simulink library "lib_fuel_converter3"  (Simulink 10.1)
settings: Solver=VariableStepAuto  StartTime=0.0  StopTime=10.0  RelTol=1e-3
undefined symbols (not defined in the file or in its folder): air_cp, amb_tmp, cyc_mph, ex_gas_cp, fc_acc_mass, fc_base_mass, fc_c2i_th_cond, fc_c_init_tmp, fc_cl2h_eff, fc_CO2_to_FUELgps, fc_cold, fc_cold_tmp, fc_cp, fc_ct_trq, fc_emisv, fc_ext_sarea, fc_fuel_den, fc_fuel_lhv, fc_h2x_th_cond, fc_h_air_flow, fc_h_cp, fc_h_init_tmp, fc_hood_emisv, fc_hood_sarea, fc_i2x_th_cond, fc_i_init_tmp, fc_inertia, fc_map_spd, fc_map_trq, fc_max_trq, fc_pwr_scale, fc_spd_scale, fc_trq_scale, fc_tstat, fc_x_init_tmp, fd_ratio, gb_num_init, gb_ratio, pow, vc_idle_bool, vc_idle_spd, vc_key_on, veh_glider_mass, wh_radius
undefined symbols (not defined in the file): fc_co_map, fc_co_map_c2h, fc_exflow_map, fc_extmp_map, fc_fuel_map, fc_fuel_map_c2h, fc_hc_map, fc_hc_map_c2h, fc_nn_model_name, fc_nox_map, fc_nox_map_c2h, fc_o2_map, fc_pm_map, fc_pm_map_c2h, generalName, logFlag
libraries: $bdroot x4, lib_etc x4, lib_fuel_converter x2, lib_fuel_converter2 x1
(part 3 of 8)

== system lib_fuel_converter3/fuel converter  <fc> for series/Model & Interface/model ==
  torque and speed  req'd at engine  output shaft (Nm) : Inport
  Block NOTES : Subsystem
      mask Display: disp('Block\nNOTES')
  Constant : Constant
  Demux : Demux  Outputs=2
  Demux1 : Demux  Outputs=3
  Logical Operator : Logic  Operator=NOT  Inputs=1
  Memory : Memory  InitialCondition=vc_idle_spd
  Mux : Mux  Inputs=2
  Mux1 : Mux  Inputs=2
  Selector : Selector  InputPortWidth=3  IndexOptions=Index vector (dialog)  Indices=[2]  OutputSizes=1
  Switch : Switch  Threshold=eps  SaturateOnIntegerOverflow=on  InputSameDT=on
  clutch disengaged : RelationalOperator  Operator===  RndMeth=Nearest  InputSameDT=on
  enhancedToWorkspace : Subsystem  TreatAsAtomicUnit=on  mask(enhancedToWorkspace){generalName=generalName, specificName=spd_out_r, logFlag=logFlag}
      mask prompts: generalName "General Name [char-evaluated]"; specificName "Specific Name [char-literal]"; logFlag "Enable flag (1=on,0=off)"
      mask help: A wrapper for the Simulink "To Workspace" block that allows you to evaluate the name of the variable to log to workspace. This is useful to avoid the double logging errors that occur when you pull in two library models that attempt to log to the same variable.
      mask init:
      | enhancedToWsMaker
      settings: CopyFcn=breakLinkCopyFcn  ParentCloseFcn=breakLinkParCloseFcn
      mask Help:
      | <h2>Enhanced To Workspace Block</h2>
      | <h3>Parameters</h3>
      | <UL>
      | <li><b>General Name:</b> This is the more general name of the variable. Variables are saved to the workspace as <i>generalName_specificName</i>. Note that this is an evaluated variable. If you would like to type in the value directly, it must be surrounded with single quotes. Otherwise you can input the name of a variable containing a char string.</li>
      | <li><b>Specific Name:</b> This is the specific name of the variable. Note that this is input as a char literal (i.e., you don't need quotes).</li>
      | <li><b>Enable Flag:</b> This flag should have the value of 0 or 1. If 0, the variable will not be logged to the workspace. If 1, the variable will be logged. This is done so that variable logging can be turned off to improve speed.</li>
      | </ul>
      | <h3>Overview</h3>
      | <p>The enhanced to workspace block was put together to allow one to dynamically resolve variable names at run time in simulink. This is most powerful when used in conjunction with a masked subsystem to allow multiple instances of that masked subsytem to be used in the same model. The strategy is to set the generalName in the block mask which will allow the block to change the general name for all variable logging on the fly.
      | <h3>Helper Files</h3>
      | <p>Three m-files are required by the enhancedToWorkspace block. These files are located in the &lt; ADVISOR root &gt;/GUI directory :
      | <ul>
      | <li><i>enhancedToWsMaker.m</i> This file runs the mask initialization for the block</li>
      | <li><i>breakLinkCopyFcn.m</i> This file is used by the block callback when the simulink block is copied. It is necessary to break the link to the enhancedToWorkspace similar to the To Workspace block in order for it to be able to configure itself. (Try copying simulink's To Workspace block--it is impossible to make a link)</li>
      | <li><i>breakLinkParCloseFcn.m</i> This file is similar to the breakLinkCopyFcn and is used when a parent system is closed</li>
      | </ul>
      | <hr>
      | 
      | <p>Created 2003-Jan-21, Michael Patrick O'Keefe, NREL</p>
      | 
      | <!--
      | <VARDEF>
      | <H3>var_name</H3>
      | <UL>
      | <LI><B>data type</B> data type here</LI>
      | <LI><B>units</B> units here</LI>
      | <LI><B>vehicle type</B> vehicle type here</LI>
      | <LI><B>description</B> description here</LI>
      | </UL>
      | </VARDEF>
      | -->
      mask Display: disp([generalName,'_',specificName])
  enhancedToWorkspace1 : Subsystem  TreatAsAtomicUnit=on  mask(enhancedToWorkspace){generalName=generalName, specificName=trq_out_r, logFlag=logFlag}
      mask prompts: generalName "General Name [char-evaluated]"; specificName "Specific Name [char-literal]"; logFlag "Enable flag (1=on,0=off)"
      mask help: A wrapper for the Simulink "To Workspace" block that allows you to evaluate the name of the variable to log to workspace. This is useful to avoid the double logging errors that occur when you pull in two library models that attempt to log to the same variable.
      mask init:
      | enhancedToWsMaker
      settings: CopyFcn=breakLinkCopyFcn  ParentCloseFcn=breakLinkParCloseFcn
      mask Help:
      | <h2>Enhanced To Workspace Block</h2>
      | <h3>Parameters</h3>
      | <UL>
      | <li><b>General Name:</b> This is the more general name of the variable. Variables are saved to the workspace as <i>generalName_specificName</i>. Note that this is an evaluated variable. If you would like to type in the value directly, it must be surrounded with single quotes. Otherwise you can input the name of a variable containing a char string.</li>
      | <li><b>Specific Name:</b> This is the specific name of the variable. Note that this is input as a char literal (i.e., you don't need quotes).</li>
      | <li><b>Enable Flag:</b> This flag should have the value of 0 or 1. If 0, the variable will not be logged to the workspace. If 1, the variable will be logged. This is done so that variable logging can be turned off to improve speed.</li>
      | </ul>
      | <h3>Overview</h3>
      | <p>The enhanced to workspace block was put together to allow one to dynamically resolve variable names at run time in simulink. This is most powerful when used in conjunction with a masked subsystem to allow multiple instances of that masked subsytem to be used in the same model. The strategy is to set the generalName in the block mask which will allow the block to change the general name for all variable logging on the fly.
      | <h3>Helper Files</h3>
      | <p>Three m-files are required by the enhancedToWorkspace block. These files are located in the &lt; ADVISOR root &gt;/GUI directory :
      | <ul>
      | <li><i>enhancedToWsMaker.m</i> This file runs the mask initialization for the block</li>
      | <li><i>breakLinkCopyFcn.m</i> This file is used by the block callback when the simulink block is copied. It is necessary to break the link to the enhancedToWorkspace similar to the To Workspace block in order for it to be able to configure itself. (Try copying simulink's To Workspace block--it is impossible to make a link)</li>
      | <li><i>breakLinkParCloseFcn.m</i> This file is similar to the breakLinkCopyFcn and is used when a parent system is closed</li>
      | </ul>
      | <hr>
      | 
      | <p>Created 2003-Jan-21, Michael Patrick O'Keefe, NREL</p>
      | 
      | <!--
      | <VARDEF>
      | <H3>var_name</H3>
      | <UL>
      | <LI><B>data type</B> data type here</LI>
      | <LI><B>units</B> units here</LI>
      | <LI><B>vehicle type</B> vehicle type here</LI>
      | <LI><B>description</B> description here</LI>
      | </UL>
      | </VARDEF>
      | -->
      mask Display: disp([generalName,'_',specificName])
  enhancedToWorkspace2 : Subsystem  TreatAsAtomicUnit=on  mask(enhancedToWorkspace){generalName=generalName, specificName=spd_est, logFlag=logFlag}
      mask prompts: generalName "General Name [char-evaluated]"; specificName "Specific Name [char-literal]"; logFlag "Enable flag (1=on,0=off)"
      mask help: A wrapper for the Simulink "To Workspace" block that allows you to evaluate the name of the variable to log to workspace. This is useful to avoid the double logging errors that occur when you pull in two library models that attempt to log to the same variable.
      mask init:
      | enhancedToWsMaker
      settings: CopyFcn=breakLinkCopyFcn  ParentCloseFcn=breakLinkParCloseFcn
      mask Help:
      | <h2>Enhanced To Workspace Block</h2>
      | <h3>Parameters</h3>
      | <UL>
      | <li><b>General Name:</b> This is the more general name of the variable. Variables are saved to the workspace as <i>generalName_specificName</i>. Note that this is an evaluated variable. If you would like to type in the value directly, it must be surrounded with single quotes. Otherwise you can input the name of a variable containing a char string.</li>
      | <li><b>Specific Name:</b> This is the specific name of the variable. Note that this is input as a char literal (i.e., you don't need quotes).</li>
      | <li><b>Enable Flag:</b> This flag should have the value of 0 or 1. If 0, the variable will not be logged to the workspace. If 1, the variable will be logged. This is done so that variable logging can be turned off to improve speed.</li>
      | </ul>
      | <h3>Overview</h3>
      | <p>The enhanced to workspace block was put together to allow one to dynamically resolve variable names at run time in simulink. This is most powerful when used in conjunction with a masked subsystem to allow multiple instances of that masked subsytem to be used in the same model. The strategy is to set the generalName in the block mask which will allow the block to change the general name for all variable logging on the fly.
      | <h3>Helper Files</h3>
      | <p>Three m-files are required by the enhancedToWorkspace block. These files are located in the &lt; ADVISOR root &gt;/GUI directory :
      | <ul>
      | <li><i>enhancedToWsMaker.m</i> This file runs the mask initialization for the block</li>
      | <li><i>breakLinkCopyFcn.m</i> This file is used by the block callback when the simulink block is copied. It is necessary to break the link to the enhancedToWorkspace similar to the To Workspace block in order for it to be able to configure itself. (Try copying simulink's To Workspace block--it is impossible to make a link)</li>
      | <li><i>breakLinkParCloseFcn.m</i> This file is similar to the breakLinkCopyFcn and is used when a parent system is closed</li>
      | </ul>
      | <hr>
      | 
      | <p>Created 2003-Jan-21, Michael Patrick O'Keefe, NREL</p>
      | 
      | <!--
      | <VARDEF>
      | <H3>var_name</H3>
      | <UL>
      | <LI><B>data type</B> data type here</LI>
      | <LI><B>units</B> units here</LI>
      | <LI><B>vehicle type</B> vehicle type here</LI>
      | <LI><B>description</B> description here</LI>
      | </UL>
      | </VARDEF>
      | -->
      mask Display: disp([generalName,'_',specificName])
  enhancedToWorkspace3 : Subsystem  TreatAsAtomicUnit=on  mask(enhancedToWorkspace){generalName=generalName, specificName=brake_trq, logFlag=logFlag}
      mask prompts: generalName "General Name [char-evaluated]"; specificName "Specific Name [char-literal]"; logFlag "Enable flag (1=on,0=off)"
      mask help: A wrapper for the Simulink "To Workspace" block that allows you to evaluate the name of the variable to log to workspace. This is useful to avoid the double logging errors that occur when you pull in two library models that attempt to log to the same variable.
      mask init:
      | enhancedToWsMaker
      settings: CopyFcn=breakLinkCopyFcn  ParentCloseFcn=breakLinkParCloseFcn
      mask Help:
      | <h2>Enhanced To Workspace Block</h2>
      | <h3>Parameters</h3>
      | <UL>
      | <li><b>General Name:</b> This is the more general name of the variable. Variables are saved to the workspace as <i>generalName_specificName</i>. Note that this is an evaluated variable. If you would like to type in the value directly, it must be surrounded with single quotes. Otherwise you can input the name of a variable containing a char string.</li>
      | <li><b>Specific Name:</b> This is the specific name of the variable. Note that this is input as a char literal (i.e., you don't need quotes).</li>
      | <li><b>Enable Flag:</b> This flag should have the value of 0 or 1. If 0, the variable will not be logged to the workspace. If 1, the variable will be logged. This is done so that variable logging can be turned off to improve speed.</li>
      | </ul>
      | <h3>Overview</h3>
      | <p>The enhanced to workspace block was put together to allow one to dynamically resolve variable names at run time in simulink. This is most powerful when used in conjunction with a masked subsystem to allow multiple instances of that masked subsytem to be used in the same model. The strategy is to set the generalName in the block mask which will allow the block to change the general name for all variable logging on the fly.
      | <h3>Helper Files</h3>
      | <p>Three m-files are required by the enhancedToWorkspace block. These files are located in the &lt; ADVISOR root &gt;/GUI directory :
      | <ul>
      | <li><i>enhancedToWsMaker.m</i> This file runs the mask initialization for the block</li>
      | <li><i>breakLinkCopyFcn.m</i> This file is used by the block callback when the simulink block is copied. It is necessary to break the link to the enhancedToWorkspace similar to the To Workspace block in order for it to be able to configure itself. (Try copying simulink's To Workspace block--it is impossible to make a link)</li>
      | <li><i>breakLinkParCloseFcn.m</i> This file is similar to the breakLinkCopyFcn and is used when a parent system is closed</li>
      | </ul>
      | <hr>
      | 
      | <p>Created 2003-Jan-21, Michael Patrick O'Keefe, NREL</p>
      | 
      | <!--
      | <VARDEF>
      | <H3>var_name</H3>
      | <UL>
      | <LI><B>data type</B> data type here</LI>
      | <LI><B>units</B> units here</LI>
      | <LI><B>vehicle type</B> vehicle type here</LI>
      | <LI><B>description</B> description here</LI>
      | </UL>
      | </VARDEF>
      | -->
      mask Display: disp([generalName,'_',specificName])
  fuel use and EO emis Configurable Subsystem : Subsystem  BlockChoice=fuel use and EO emis
      link override fuel use and EO emis/enhancedToWorkspace1/To Workspace: VariableName=fc_th_pwr  SampleTime=-1  SaveFormat=Array
      link override fuel use and EO emis/enhancedToWorkspace10/To Workspace: VariableName=fc_ex_gas_tmp  SampleTime=-1  SaveFormat=Array
      link override fuel use and EO emis/enhancedToWorkspace11/To Workspace: VariableName=fc_ex_th_pwr  SampleTime=-1  SaveFormat=Array
      link override fuel use and EO emis/enhancedToWorkspace12/To Workspace: VariableName=fc_clt_tmp  SampleTime=-1  SaveFormat=Array
      link override fuel use and EO emis/enhancedToWorkspace2/To Workspace: VariableName=fc_o2_flow  SampleTime=-1  SaveFormat=Array
      link override fuel use and EO emis/enhancedToWorkspace3/To Workspace: VariableName=fc_r_th_pwr  SampleTime=-1  SaveFormat=Array
      link override fuel use and EO emis/enhancedToWorkspace5/To Workspace: VariableName=fc_h_th_pwr  SampleTime=-1  SaveFormat=Array
      link override fuel use and EO emis/enhancedToWorkspace6/To Workspace: VariableName=fc_tmp  SampleTime=-1  SaveFormat=Array
      link override fuel use and EO emis/enhancedToWorkspace7/To Workspace: VariableName=fc_fuel_rate  SampleTime=-1  SaveFormat=Array
      link override fuel use and EO emis/enhancedToWorkspace8/To Workspace: VariableName=fc_emis_eo  SampleTime=-1  SaveFormat=Array
      link override fuel use and EO emis/enhancedToWorkspace9/To Workspace: VariableName=fc_ex_gas_flow  SampleTime=-1  SaveFormat=Array
      settings: AttributesFormatString=%<BlockChoice>  TemplateBlock=lib_fuel_converter3/configurable subsystems/fuel use and EO emis Configurable Subsystem  MemberBlocks=fuel use and EO emis,fuel use and EO emis Neural Network Model
  help : Subsystem
      settings: OpenFcn=web(['file:\\\' which('fuel_converter.htm')]);
      mask Display: image(imread('doc_man.jpg'))
  providing trq (+ive or -ive) : Subsystem
  spinning up or spinning down : Subsystem
  fuel use : Outport  InitialOutput=0
  EO emis info : Outport  Port=2  InitialOutput=0
  "torque and speed  avail. to driveline (Nm), (rad/s)" : Outport  Port=3  InitialOutput=0
  tag scope: engine_speed=scoped, fc_brake_trq=scoped, fc_spd_est=scoped, fc_spd_out_a=scoped, fc_spd_out_r=scoped, fc_trq_out_a=scoped, fc_trq_out_r=scoped, fuel=scoped
  wires:
  Selector/1 -> [fc_spd_est], enhancedToWorkspace2/1(In1)
  fuel use and EO emis Configurable Subsystem/1(cumulative fuel  use (gal)) -> [fuel], fuel use/1
  Switch/1 -> Demux1/1
  Memory/1 -> providing trq (+ive or -ive)/3(prev engine spd (rad/s)), spinning up or spinning down/3(previous engine spd (rad/s))
  spinning up or spinning down/1(map trq (Nm) spd (rad/s) trq to drivetrain (Nm)) -> Switch/3
  providing trq (+ive or -ive)/1(map trq (Nm) spd (rad/s) trq to drivetrain (Nm)) -> Selector/1, Switch/1
  Logical Operator/1 -> Switch/2
  [clutch_state] -> clutch disengaged/2
  Constant/1 -> clutch disengaged/1
  clutch disengaged/1 -> Logical Operator/1, spinning up or spinning down/2(engine disconnected from drivetrain)
  Demux/2 -> [fc_spd_out_r], enhancedToWorkspace/1(In1), spinning up or spinning down/1(spd command (rad/s)), providing trq (+ive or -ive)/2(req'd spd (rad/s))
  Demux/1 -> providing trq (+ive or -ive)/1(req'd trq (Nm)), [fc_trq_out_r], enhancedToWorkspace1/1(In1)
  torque and speed  req'd at engine  output shaft (Nm)/1 -> Demux/1
  Demux1/1 -> fuel use and EO emis Configurable Subsystem/1(T (Nm)), [fc_brake_trq], enhancedToWorkspace3/1(In1)
  Demux1/3 -> [fc_trq_out_a], Mux1/1
  Demux1/2 -> fuel use and EO emis Configurable Subsystem/2(w (rad/s)), Mux1/2, Memory/1, [fc_spd_out_a], [engine_speed]
  Mux/1 -> EO emis info/1
  fuel use and EO emis Configurable Subsystem/2("FC ON?, EOem, MFex, Tex, O2ex") -> Mux/1
  fuel use and EO emis Configurable Subsystem/3(Vv,Tfc) -> Mux/2
  Mux1/1 -> "torque and speed  avail. to driveline (Nm), (rad/s)"/1

== system lib_fuel_converter3/fuel converter  <fc> for series/Model & Interface/signal annotator ==
  In1 : Inport
  Demux : Demux  Outputs=2
  Mux : Mux  Inputs=2
  Out1 : Outport
  wires:
  Mux/1 -> Out1/1
  In1/1 -> Demux/1
  Demux/1 -> Mux/1  "fc_trq_out_r"
  Demux/2 -> Mux/2  "fc_spd_out_r"

== system lib_fuel_converter3/fuel converter <fc>/IC Engine Model  &  Interface/ic engine model ==
  torque and speed  req'd at engine  output shaft (Nm) : Inport
  Block NOTES : Subsystem
      mask Display: disp('Block\nNOTES')
  Demux : Demux  Outputs=2
  Mux : Mux  Inputs=2
  Mux1 : Mux  Inputs=2
  Speed Limits : Subsystem
  engine speed estimator : Subsystem
  engine torque : Subsystem
  enhancedToWorkspace : Subsystem  mask(enhancedToWorkspace){generalName=generalName, specificName=spd_out_r, logFlag=logFlag}
      mask prompts: generalName "General Name [char-evaluated]"; specificName "Specific Name [char-literal]"; logFlag "Enable flag (1=on,0=off)"
      mask help: A wrapper for the Simulink "To Workspace" block that allows you to evaluate the name of the variable to log to workspace. This is useful to avoid the double logging errors that occur when you pull in two library models that attempt to log to the same variable.
      mask init:
      | enhancedToWsMaker
      settings: CopyFcn=breakLinkCopyFcn
      mask Display: disp([generalName,'_',specificName])
  enhancedToWorkspace1 : Subsystem  mask(enhancedToWorkspace){generalName=generalName, specificName=spd_est, logFlag=logFlag}
      mask prompts: generalName "General Name [char-evaluated]"; specificName "Specific Name [char-literal]"; logFlag "Enable flag (1=on,0=off)"
      mask help: A wrapper for the Simulink "To Workspace" block that allows you to evaluate the name of the variable to log to workspace. This is useful to avoid the double logging errors that occur when you pull in two library models that attempt to log to the same variable.
      mask init:
      | enhancedToWsMaker
      settings: CopyFcn=breakLinkCopyFcn
      mask Display: disp([generalName,'_',specificName])
  enhancedToWorkspace3 : Subsystem  mask(enhancedToWorkspace){generalName=generalName, specificName=fuel, logFlag=logFlag}
      mask prompts: generalName "General Name [char-evaluated]"; specificName "Specific Name [char-literal]"; logFlag "Enable flag (1=on,0=off)"
      mask help: A wrapper for the Simulink "To Workspace" block that allows you to evaluate the name of the variable to log to workspace. This is useful to avoid the double logging errors that occur when you pull in two library models that attempt to log to the same variable.
      mask init:
      | enhancedToWsMaker
      settings: CopyFcn=breakLinkCopyFcn
      mask Display: disp([generalName,'_',specificName])
  enhancedToWorkspace4 : Subsystem  mask(enhancedToWorkspace){generalName=generalName, specificName=spd_out_a, logFlag=logFlag}
      mask prompts: generalName "General Name [char-evaluated]"; specificName "Specific Name [char-literal]"; logFlag "Enable flag (1=on,0=off)"
      mask help: A wrapper for the Simulink "To Workspace" block that allows you to evaluate the name of the variable to log to workspace. This is useful to avoid the double logging errors that occur when you pull in two library models that attempt to log to the same variable.
      mask init:
      | enhancedToWsMaker
      settings: CopyFcn=breakLinkCopyFcn
      mask Display: disp([generalName,'_',specificName])
  enhancedToWorkspace5 : Subsystem  mask(enhancedToWorkspace){generalName=generalName, specificName=trq_out_a, logFlag=logFlag}
      mask prompts: generalName "General Name [char-evaluated]"; specificName "Specific Name [char-literal]"; logFlag "Enable flag (1=on,0=off)"
      mask help: A wrapper for the Simulink "To Workspace" block that allows you to evaluate the name of the variable to log to workspace. This is useful to avoid the double logging errors that occur when you pull in two library models that attempt to log to the same variable.
      mask init:
      | enhancedToWsMaker
      settings: CopyFcn=breakLinkCopyFcn
      mask Display: disp([generalName,'_',specificName])
  enhancedToWorkspace6 : Subsystem  mask(enhancedToWorkspace){generalName=generalName, specificName=trq_out_r, logFlag=logFlag}
      mask prompts: generalName "General Name [char-evaluated]"; specificName "Specific Name [char-literal]"; logFlag "Enable flag (1=on,0=off)"
      mask help: A wrapper for the Simulink "To Workspace" block that allows you to evaluate the name of the variable to log to workspace. This is useful to avoid the double logging errors that occur when you pull in two library models that attempt to log to the same variable.
      mask init:
      | enhancedToWsMaker
      settings: CopyFcn=breakLinkCopyFcn
      mask Display: disp([generalName,'_',specificName])
  enhancedToWorkspace7 : Subsystem  mask(enhancedToWorkspace){generalName=generalName, specificName=brake_trq, logFlag=logFlag}
      mask prompts: generalName "General Name [char-evaluated]"; specificName "Specific Name [char-literal]"; logFlag "Enable flag (1=on,0=off)"
      mask help: A wrapper for the Simulink "To Workspace" block that allows you to evaluate the name of the variable to log to workspace. This is useful to avoid the double logging errors that occur when you pull in two library models that attempt to log to the same variable.
      mask init:
      | enhancedToWsMaker
      settings: CopyFcn=breakLinkCopyFcn
      mask Display: disp([generalName,'_',specificName])
  fuel use and EO emis Configurable Subsystem : Subsystem  BlockChoice=fuel use and EO emis
      link override fuel use and EO emis/enhancedToWorkspace1/To Workspace: VariableName=fc_th_pwr  SampleTime=-1  SaveFormat=Array
      link override fuel use and EO emis/enhancedToWorkspace10/To Workspace: VariableName=fc_ex_gas_tmp  SampleTime=-1  SaveFormat=Array
      link override fuel use and EO emis/enhancedToWorkspace11/To Workspace: VariableName=fc_ex_th_pwr  SampleTime=-1  SaveFormat=Array
      link override fuel use and EO emis/enhancedToWorkspace12/To Workspace: VariableName=fc_clt_tmp  SampleTime=-1  SaveFormat=Array
      link override fuel use and EO emis/enhancedToWorkspace2/To Workspace: VariableName=fc_o2_flow  SampleTime=-1  SaveFormat=Array
      link override fuel use and EO emis/enhancedToWorkspace3/To Workspace: VariableName=fc_r_th_pwr  SampleTime=-1  SaveFormat=Array
      link override fuel use and EO emis/enhancedToWorkspace5/To Workspace: VariableName=fc_h_th_pwr  SampleTime=-1  SaveFormat=Array
      link override fuel use and EO emis/enhancedToWorkspace6/To Workspace: VariableName=fc_tmp  SampleTime=-1  SaveFormat=Array
      link override fuel use and EO emis/enhancedToWorkspace7/To Workspace: VariableName=fc_fuel_rate  SampleTime=-1  SaveFormat=Array
      link override fuel use and EO emis/enhancedToWorkspace8/To Workspace: VariableName=fc_emis_eo  SampleTime=-1  SaveFormat=Array
      link override fuel use and EO emis/enhancedToWorkspace9/To Workspace: VariableName=fc_ex_gas_flow  SampleTime=-1  SaveFormat=Array
      settings: AttributesFormatString=%<BlockChoice>  TemplateBlock=lib_fuel_converter3/configurable subsystems/fuel use and EO emis Configurable Subsystem  MemberBlocks=fuel use and EO emis,fuel use and EO emis Neural Network Model
  help : Subsystem
      settings: OpenFcn=web(['file:\\\' which('fuel_converter.htm')]);
      mask Display: image(imread('doc_man.jpg'))
  fuel use : Outport  InitialOutput=0
  EO emis info : Outport  Port=2  InitialOutput=0
  "torque and speed  avail. to driveline (Nm), (rad/s)" : Outport  Port=3  InitialOutput=0
  tag scope: fc_spd_est=scoped, fc_spd_out_a=scoped, fc_spd_out_r=scoped, fc_trq_out_a=scoped, fuel=scoped
  wires:
  engine torque/2(torque to shaft (Nm)) -> [fc_trq_out_a], Mux1/1, enhancedToWorkspace5/1(In1)
  engine torque/1(map torque (Nm)) -> enhancedToWorkspace7/1(In1), fuel use and EO emis Configurable Subsystem/1(T (Nm))
  Mux1/1 -> "torque and speed  avail. to driveline (Nm), (rad/s)"/1
  fuel use and EO emis Configurable Subsystem/3(Vv,Tfc) -> Mux/2
  fuel use and EO emis Configurable Subsystem/2("FC ON?, EOem, MFex, Tex, O2ex") -> Mux/1
  Mux/1 -> EO emis info/1
  Demux/1 -> engine torque/1(fc_trq_out_r), enhancedToWorkspace6/1(In1)
  torque and speed  req'd at engine  output shaft (Nm)/1 -> Demux/1
  Demux/2 -> Speed Limits/1(Speed Requested), [fc_spd_out_r], enhancedToWorkspace/1(In1)
  fuel use and EO emis Configurable Subsystem/1(cumulative fuel  use (gal)) -> fuel use/1, [fuel], enhancedToWorkspace3/1(In1)
  engine speed estimator/1(Out1) -> engine torque/3(engine spd), fuel use and EO emis Configurable Subsystem/2(w (rad/s)), [fc_spd_est], enhancedToWorkspace1/1(In1)
  Speed Limits/1(Limited Speed Request) -> engine torque/2(spd command), engine speed estimator/1(spd command), Mux1/2, [fc_spd_out_a], enhancedToWorkspace4/1(In1)

== system lib_fuel_converter3/fuel converter <fc>/IC Engine Model  &  Interface/signal annotator ==
  In1 : Inport
  Demux : Demux  Outputs=2
  Mux : Mux  Inputs=1
  Terminator : Terminator
  Out1 : Outport
  tag scope: fc_trq_out_r=scoped
  wires:
  Mux/1 -> Out1/1
  [fc_spd_est] -> Mux/1  "fc_spd_est"
  In1/1 -> Demux/1
  Demux/1 -> [fc_trq_out_r]  "fc_trq_out_r"
  Demux/2 -> Terminator/1  "fc_spd_out_r"

== system lib_fuel_converter3/fuel converter <fc> no fuel at negative torque/IC Engine Model  &  Interface/ic engine model ==
  torque and speed  req'd at engine  output shaft (Nm) : Inport
  Block NOTES : Subsystem
      mask Display: disp('Block\nNOTES')
  Demux : Demux  Outputs=2
  Demux1 : Demux  Outputs=2
  Demux2 : Demux  Outputs=2
  Mux : Mux  Inputs=2
  Mux1 : Mux  Inputs=2
  Speed Limits : Subsystem
  achieved power and energy : Subsystem
  engine speed estimator : Subsystem
  engine torque : Subsystem
  enhancedToWorkspace : Subsystem  mask(enhancedToWorkspace){generalName=generalName, specificName=spd_out_r, logFlag=logFlag}
      mask prompts: generalName "General Name [char-evaluated]"; specificName "Specific Name [char-literal]"; logFlag "Enable flag (1=on,0=off)"
      mask help: A wrapper for the Simulink "To Workspace" block that allows you to evaluate the name of the variable to log to workspace. This is useful to avoid the double logging errors that occur when you pull in two library models that attempt to log to the same variable.
      mask init:
      | enhancedToWsMaker
      settings: CopyFcn=breakLinkCopyFcn
      mask Display: disp([generalName,'_',specificName])
  enhancedToWorkspace1 : Subsystem  mask(enhancedToWorkspace){generalName=generalName, specificName=spd_est, logFlag=logFlag}
      mask prompts: generalName "General Name [char-evaluated]"; specificName "Specific Name [char-literal]"; logFlag "Enable flag (1=on,0=off)"
      mask help: A wrapper for the Simulink "To Workspace" block that allows you to evaluate the name of the variable to log to workspace. This is useful to avoid the double logging errors that occur when you pull in two library models that attempt to log to the same variable.
      mask init:
      | enhancedToWsMaker
      settings: CopyFcn=breakLinkCopyFcn
      mask Display: disp([generalName,'_',specificName])
  enhancedToWorkspace3 : Subsystem  mask(enhancedToWorkspace){generalName=generalName, specificName=fuel, logFlag=logFlag}
      mask prompts: generalName "General Name [char-evaluated]"; specificName "Specific Name [char-literal]"; logFlag "Enable flag (1=on,0=off)"
      mask help: A wrapper for the Simulink "To Workspace" block that allows you to evaluate the name of the variable to log to workspace. This is useful to avoid the double logging errors that occur when you pull in two library models that attempt to log to the same variable.
      mask init:
      | enhancedToWsMaker
      settings: CopyFcn=breakLinkCopyFcn
      mask Display: disp([generalName,'_',specificName])
  enhancedToWorkspace4 : Subsystem  mask(enhancedToWorkspace){generalName=generalName, specificName=spd_out_a, logFlag=logFlag}
      mask prompts: generalName "General Name [char-evaluated]"; specificName "Specific Name [char-literal]"; logFlag "Enable flag (1=on,0=off)"
      mask help: A wrapper for the Simulink "To Workspace" block that allows you to evaluate the name of the variable to log to workspace. This is useful to avoid the double logging errors that occur when you pull in two library models that attempt to log to the same variable.
      mask init:
      | enhancedToWsMaker
      settings: CopyFcn=breakLinkCopyFcn
      mask Display: disp([generalName,'_',specificName])
  enhancedToWorkspace5 : Subsystem  mask(enhancedToWorkspace){generalName=generalName, specificName=trq_out_a, logFlag=logFlag}
      mask prompts: generalName "General Name [char-evaluated]"; specificName "Specific Name [char-literal]"; logFlag "Enable flag (1=on,0=off)"
      mask help: A wrapper for the Simulink "To Workspace" block that allows you to evaluate the name of the variable to log to workspace. This is useful to avoid the double logging errors that occur when you pull in two library models that attempt to log to the same variable.
      mask init:
      | enhancedToWsMaker
      settings: CopyFcn=breakLinkCopyFcn
      mask Display: disp([generalName,'_',specificName])
  enhancedToWorkspace6 : Subsystem  mask(enhancedToWorkspace){generalName=generalName, specificName=trq_out_r, logFlag=logFlag}
      mask prompts: generalName "General Name [char-evaluated]"; specificName "Specific Name [char-literal]"; logFlag "Enable flag (1=on,0=off)"
      mask help: A wrapper for the Simulink "To Workspace" block that allows you to evaluate the name of the variable to log to workspace. This is useful to avoid the double logging errors that occur when you pull in two library models that attempt to log to the same variable.
      mask init:
      | enhancedToWsMaker
      settings: CopyFcn=breakLinkCopyFcn
      mask Display: disp([generalName,'_',specificName])
  enhancedToWorkspace7 : Subsystem  mask(enhancedToWorkspace){generalName=generalName, specificName=brake_trq, logFlag=logFlag}
      mask prompts: generalName "General Name [char-evaluated]"; specificName "Specific Name [char-literal]"; logFlag "Enable flag (1=on,0=off)"
      mask help: A wrapper for the Simulink "To Workspace" block that allows you to evaluate the name of the variable to log to workspace. This is useful to avoid the double logging errors that occur when you pull in two library models that attempt to log to the same variable.
      mask init:
      | enhancedToWsMaker
      settings: CopyFcn=breakLinkCopyFcn
      mask Display: disp([generalName,'_',specificName])
  fuel use and EO emis no fuel used at negative torque : Subsystem
  help : Subsystem
      settings: OpenFcn=web(['file:\\\' which('fuel_converter.htm')]);
      mask Display: image(imread('doc_man.jpg'))
  requested power and energy : Subsystem
  fuel use : Outport  InitialOutput=0
  EO emis info : Outport  Port=2  InitialOutput=0
  "torque and speed  avail. to driveline (Nm), (rad/s)" : Outport  Port=3  InitialOutput=0
  tag scope: fc_spd_est=scoped, fc_spd_out_a=scoped, fc_spd_out_r=scoped, fc_trq_out_a=scoped, fuel=scoped
  wires:
  engine torque/2(torque to shaft (Nm)) -> [fc_trq_out_a], Mux1/1, enhancedToWorkspace5/1(In1)
  engine torque/1(map torque (Nm)) -> enhancedToWorkspace7/1(In1), fuel use and EO emis no fuel used at negative torque/1(T (Nm))
  Mux1/1 -> "torque and speed  avail. to driveline (Nm), (rad/s)"/1, Demux2/1
  fuel use and EO emis no fuel used at negative torque/3(Vv,Tfc) -> Mux/2
  fuel use and EO emis no fuel used at negative torque/2("FC ON?, EOem, MFex, Tex, O2ex") -> Mux/1
  Mux/1 -> EO emis info/1
  Demux/1 -> engine torque/1(fc_trq_out_r), enhancedToWorkspace6/1(In1)
  torque and speed  req'd at engine  output shaft (Nm)/1 -> Demux/1, Demux1/1
  Demux/2 -> Speed Limits/1(Speed Requested), [fc_spd_out_r], enhancedToWorkspace/1(In1)
  fuel use and EO emis no fuel used at negative torque/1(cumulative fuel  use (gal)) -> fuel use/1, [fuel], enhancedToWorkspace3/1(In1)
  engine speed estimator/1(Out1) -> engine torque/3(engine spd), fuel use and EO emis no fuel used at negative torque/2(w (rad/s)), [fc_spd_est], enhancedToWorkspace1/1(In1)
  Speed Limits/1(Limited Speed Request) -> engine torque/2(spd command), engine speed estimator/1(spd command), Mux1/2, [fc_spd_out_a], enhancedToWorkspace4/1(In1)
  Demux1/1 -> requested power and energy/1(trq)
  Demux1/2 -> requested power and energy/2(spd)
  Demux2/1 -> achieved power and energy/1(trq)
  Demux2/2 -> achieved power and energy/2(spd)

== system lib_fuel_converter3/fuel converter <fc> no fuel at negative torque/IC Engine Model  &  Interface/signal annotator ==
  In1 : Inport
  Demux : Demux  Outputs=2
  Mux : Mux  Inputs=3
  Out1 : Outport
  wires:
  [fc_spd_est] -> Mux/3  "fc_spd_est"
  In1/1 -> Demux/1
  Demux/1 -> Mux/1  "fc_trq_out_r"
  Demux/2 -> Mux/2  "fc_spd_out_r"
  Mux/1 -> Out1/1

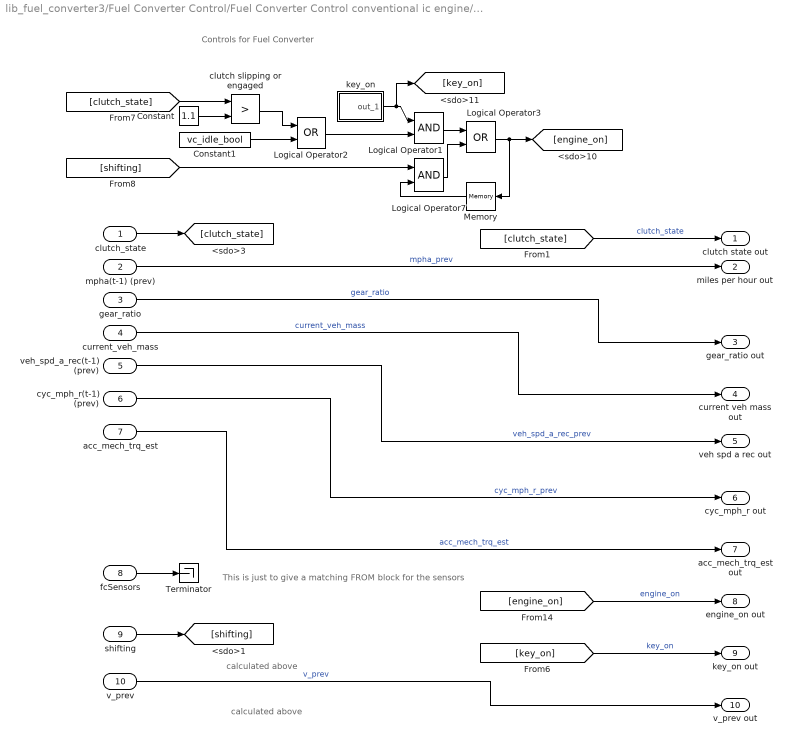
== system lib_fuel_converter3/Fuel Converter Control/Fuel Converter Control conventional ic engine/conventional IC engine/Fuel Converter Control ==
  note: Controls for Fuel Converter
  note: This is just to give a matching FROM block for the sensors
  note: calculated above
  note: calculated above
  clutch_state : Inport
  mpha(t-1) (prev) : Inport  Port=2
  gear_ratio : Inport  Port=3
  current_veh_mass : Inport  Port=4
  veh_spd_a_rec(t-1) (prev) : Inport  Port=5
  cyc_mph_r(t-1) (prev) : Inport  Port=6
  acc_mech_trq_est : Inport  Port=7
  fcSensors : Inport  Port=8
  shifting : Inport  Port=9
  v_prev : Inport  Port=10
  Constant : Constant  Value=1.1
  Constant1 : Constant  Value=vc_idle_bool
  Logical Operator1 : Logic
  Logical Operator2 : Logic  Operator=OR
  Logical Operator3 : Logic  Operator=OR
  Logical Operator7 : Logic
  Memory : Memory
  Terminator : Terminator
  clutch slipping or engaged : RelationalOperator  Operator=>  RndMeth=Nearest  InputSameDT=on
  key_on : Subsystem  mask(Repeating table){Parameter1=vc_key_on(:,1), Parameter2=vc_key_on(:,2)}
      mask prompts: Parameter1 "Time values:"; Parameter2 "Output values:"
      mask help:
      | Repeating table.
      | Enter values of time and output for first cycle.
      mask init:
      | period = max(@1); t = @1; y = @2;
      mask Help: Repeats cycle given in table. Time values should be monotonically increasing.
  clutch state out : Outport
  miles per hour out : Outport  Port=2
  gear_ratio out : Outport  Port=3
  current veh mass out : Outport  Port=4
  veh spd a rec out : Outport  Port=5
  cyc_mph_r out : Outport  Port=6
  acc_mech_trq_est out : Outport  Port=7
  engine_on out : Outport  Port=8
  key_on out : Outport  Port=9
  v_prev out : Outport  Port=10
  wires:
  gear_ratio/1 -> gear_ratio out/1  "gear_ratio"
  [clutch_state] -> clutch slipping or engaged/1
  Constant1/1 -> Logical Operator2/2
  Constant/1 -> clutch slipping or engaged/2
  clutch slipping or engaged/1 -> Logical Operator2/1
  Logical Operator1/1 -> Logical Operator3/1
  Logical Operator2/1 -> Logical Operator1/2
  [shifting] -> Logical Operator7/1
  Memory/1 -> Logical Operator7/2
  Logical Operator7/1 -> Logical Operator3/2
  Logical Operator3/1 -> [engine_on], Memory/1
  key_on/1(out_1) -> Logical Operator1/1, [key_on]
  fcSensors/1 -> Terminator/1
  shifting/1 -> [shifting]
  clutch_state/1 -> [clutch_state]
  mpha(t-1) (prev)/1 -> miles per hour out/1  "mpha_prev"
  current_veh_mass/1 -> current veh mass out/1  "current_veh_mass"
  veh_spd_a_rec(t-1) (prev)/1 -> veh spd a rec out/1  "veh_spd_a_rec_prev"
  cyc_mph_r(t-1) (prev)/1 -> cyc_mph_r out/1  "cyc_mph_r_prev"
  acc_mech_trq_est/1 -> acc_mech_trq_est out/1  "acc_mech_trq_est"
  v_prev/1 -> v_prev out/1  "v_prev"
  [clutch_state] -> clutch state out/1  "clutch_state"
  [engine_on] -> engine_on out/1  "engine_on"
  [key_on] -> key_on out/1  "key_on"

== system lib_fuel_converter3/configurable subsystems/fuel use and EO emis/HOT engine maps/Block NOTES ==
  note: This block determines the fully hot fuel use, engine-out emissions output rates, exhaust gas mass flow rate,
      | and engine-out exhaust gas temperature as a function of engine output torque and speed.
      | The engine maps (except for exhaust gas temperature) can be scaled using variables fc_spd_scale and
      |  fc_trq_scale; it is recommended that scaling values outside the range of 0.85 to 1.15 be used CAREFULLY.

== system lib_fuel_converter3/configurable subsystems/fuel use and EO emis/HOT engine maps/CO (g/s) ==
  x0 : Inport
  y0 : Inport  Port=2
  Mux : Mux  Inputs=2
  S-function : S-Function  FunctionName=sftable2  Parameters=xindex, yindex, table  SFunctionDeploymentMode=off  EnableBusSupport=off
  table out : Outport  InitialOutput=0
  wires:
  y0/1 -> Mux/2
  S-function/1 -> table out/1
  x0/1 -> Mux/1
  Mux/1 -> S-function/1

== system lib_fuel_converter3/configurable subsystems/fuel use and EO emis/HOT engine maps/HC (g/s) ==
  x0 : Inport
  y0 : Inport  Port=2
  Mux : Mux  Inputs=2
  S-function : S-Function  FunctionName=sftable2  Parameters=xindex, yindex, table  SFunctionDeploymentMode=off  EnableBusSupport=off
  table out : Outport  InitialOutput=0
  wires:
  y0/1 -> Mux/2
  S-function/1 -> table out/1
  x0/1 -> Mux/1
  Mux/1 -> S-function/1

== system lib_fuel_converter3/configurable subsystems/fuel use and EO emis/HOT engine maps/MF,ex (g/s) ==
  x0 : Inport
  y0 : Inport  Port=2
  Mux : Mux  Inputs=2
  S-function : S-Function  FunctionName=sftable2  Parameters=xindex, yindex, table  SFunctionDeploymentMode=off  EnableBusSupport=off
  table out : Outport  InitialOutput=0
  wires:
  y0/1 -> Mux/2
  S-function/1 -> table out/1
  x0/1 -> Mux/1
  Mux/1 -> S-function/1

== system lib_fuel_converter3/configurable subsystems/fuel use and EO emis/HOT engine maps/NOx (g/s) ==
  x0 : Inport
  y0 : Inport  Port=2
  Mux : Mux  Inputs=2
  S-function : S-Function  FunctionName=sftable2  Parameters=xindex, yindex, table  SFunctionDeploymentMode=off  EnableBusSupport=off
  table out : Outport  InitialOutput=0
  wires:
  y0/1 -> Mux/2
  S-function/1 -> table out/1
  x0/1 -> Mux/1
  Mux/1 -> S-function/1

== system lib_fuel_converter3/configurable subsystems/fuel use and EO emis/HOT engine maps/O2 (g/s) ==
  x0 : Inport
  y0 : Inport  Port=2
  Mux : Mux  Inputs=2
  S-function : S-Function  FunctionName=sftable2  Parameters=xindex, yindex, table  SFunctionDeploymentMode=off  EnableBusSupport=off
  table out : Outport  InitialOutput=0
  wires:
  Mux/1 -> S-function/1
  x0/1 -> Mux/1
  S-function/1 -> table out/1
  y0/1 -> Mux/2

== system lib_fuel_converter3/configurable subsystems/fuel use and EO emis/HOT engine maps/PM (g/s) ==
  x0 : Inport
  y0 : Inport  Port=2
  Mux : Mux  Inputs=2
  S-function : S-Function  FunctionName=sftable2  Parameters=xindex, yindex, table  SFunctionDeploymentMode=off  EnableBusSupport=off
  table out : Outport  InitialOutput=0
  wires:
  y0/1 -> Mux/2
  S-function/1 -> table out/1
  x0/1 -> Mux/1
  Mux/1 -> S-function/1

== system lib_fuel_converter3/configurable subsystems/fuel use and EO emis/HOT engine maps/Tex,eo (C) ==
  x0 : Inport
  y0 : Inport  Port=2
  Mux : Mux  Inputs=2
  S-function : S-Function  FunctionName=sftable2  Parameters=xindex, yindex, table  SFunctionDeploymentMode=off  EnableBusSupport=off
  table out : Outport  InitialOutput=0
  wires:
  y0/1 -> Mux/2
  S-function/1 -> table out/1
  x0/1 -> Mux/1
  Mux/1 -> S-function/1

== system lib_fuel_converter3/configurable subsystems/fuel use and EO emis/HOT engine maps/fuel (g/s) ==
  x0 : Inport
  y0 : Inport  Port=2
  Mux : Mux  Inputs=2
  S-function : S-Function  FunctionName=sftable2  Parameters=xindex, yindex, table  SFunctionDeploymentMode=off  EnableBusSupport=off
  table out : Outport  InitialOutput=0
  wires:
  y0/1 -> Mux/2
  S-function/1 -> table out/1
  x0/1 -> Mux/1
  Mux/1 -> S-function/1

== system lib_fuel_converter3/configurable subsystems/fuel use and EO emis/fc temp/Block NOTES ==
  note: This block models the thermal behavior internal combustion engine (ICE).
      | Emphasis is on the coolant since this temperature is used to correct engine
      | fuel use.

== system lib_fuel_converter3/configurable subsystems/fuel use and EO emis/fc temp/fc coolant ==
  Tcl : Inport
  "Qfc_i " : Inport  Port=2
  Enable : EnablePort  StatesWhenEnabling=reset
  Constant : Constant  Value=fc_tstat
  Product1 : Product  SaturateOnIntegerOverflow=on
  Qhtr : Fcn  Expr=fc_cl2h_eff*fc_h_air_flow*air_cp*(u - amb_tmp)
  Qi : Sum  Inputs=-+  SaturateOnIntegerOverflow=on
  Relational Operator : RelationalOperator  Operator=<=  RndMeth=Nearest  InputSameDT=on
  Qfc_rad : Outport  OutputWhenDisabled=reset  InitialOutput=0
  Qfc_htr : Outport  Port=2  OutputWhenDisabled=reset  InitialOutput=0
  wires:
  Tcl/1 -> Qhtr/1, Relational Operator/2
  Relational Operator/1 -> Product1/1
  Constant/1 -> Relational Operator/1
  Product1/1 -> Qfc_rad/1
  "Qfc_i "/1 -> Qi/2
  Qhtr/1 -> Qi/1, Qfc_htr/1
  Qi/1 -> Product1/2

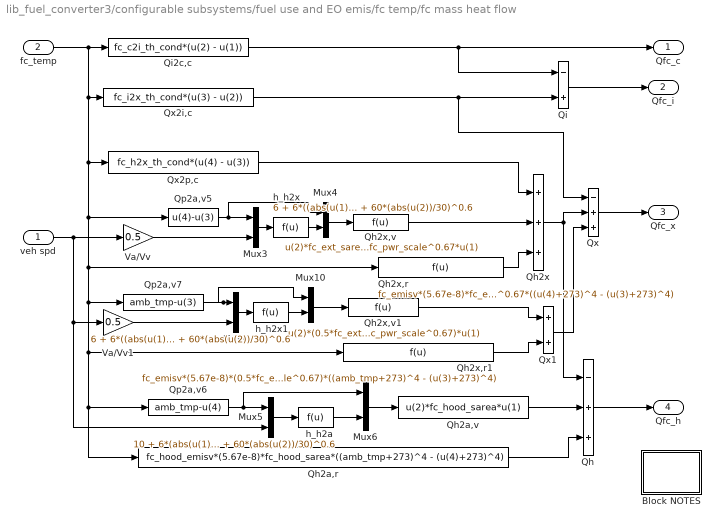
== system lib_fuel_converter3/configurable subsystems/fuel use and EO emis/fc temp/fc mass heat flow ==
  veh spd : Inport
  fc_temp : Inport  Port=2
  Block NOTES : Subsystem
      mask Display: disp('Block\nNOTES')
  Mux{3..6,9..10} (6 alike) : Mux  Inputs=2
  Qh : Sum  Inputs=-++  SaturateOnIntegerOverflow=on
  Qh2a,r : Fcn  Expr=fc_hood_emisv*(5.67e-8)*fc_hood_sarea*((amb_tmp+273)^4 - (u(4)+273)^4)
  Qh2a,v : Fcn  Expr=u(2)*fc_hood_sarea*u(1)
  Qh2x : Sum  Inputs=+++  SaturateOnIntegerOverflow=on
  Qh2x,r : Fcn  Expr=fc_emisv*(5.67e-8)*fc_ext_sarea*fc_pwr_scale^0.67*((u(4)+273)^4 - (u(3)+273)^4)
  Qh2x,r1 : Fcn  Expr=fc_emisv*(5.67e-8)*(0.5*fc_ext_sarea*fc_pwr_scale^0.67)*((amb_tmp+273)^4 - (u(3)+273)^4)
  Qh2x,v : Fcn  Expr=u(2)*fc_ext_sarea*fc_pwr_scale^0.67*u(1)
  Qh2x,v1 : Fcn  Expr=u(2)*(0.5*fc_ext_sarea*fc_pwr_scale^0.67)*u(1)
  Qi : Sum  Inputs=-+  SaturateOnIntegerOverflow=on
  Qi2c,c : Fcn  Expr=fc_c2i_th_cond*(u(2) - u(1))
  Qp2a,v5 : Fcn  Expr=u(4)-u(3)
  Qp2a,v6 : Fcn  Expr=amb_tmp-u(4)
  Qp2a,v7 : Fcn  Expr=amb_tmp-u(3)
  Qx : Sum  Inputs=-++  SaturateOnIntegerOverflow=on
  Qx1 : Sum  SaturateOnIntegerOverflow=on
  Qx2i,c : Fcn  Expr=fc_i2x_th_cond*(u(3) - u(2))
  Qx2p,c : Fcn  Expr=fc_h2x_th_cond*(u(4) - u(3))
  Va/Vv : Gain  Gain=0.5  SaturateOnIntegerOverflow=on
  Va/Vv1 : Gain  Gain=0.5  SaturateOnIntegerOverflow=on
  h_h2a : Fcn  Expr=10 + 6*(abs(u(1))/1000)^0.3 + 60*(abs(u(2))/30)^0.6
  h_h2x : Fcn  Expr=6 + 6*((abs(u(1))/1000))^0.3 + 60*(abs(u(2))/30)^0.6
  h_h2x1 : Fcn  Expr=6 + 6*((abs(u(1))/1000))^0.3 + 60*(abs(u(2))/30)^0.6
  Qfc_c : Outport
  Qfc_i : Outport  Port=2
  Qfc_x : Outport  Port=3
  Qfc_h : Outport  Port=4
  wires:
  Mux10/1 -> Qh2x,v1/1
  Mux9/1 -> h_h2x1/1
  Qp2a,v7/1 -> Mux9/1, Mux10/1
  h_h2x1/1 -> Mux10/2
  Va/Vv1/1 -> Mux9/2
  Mux4/1 -> Qh2x,v/1
  Mux3/1 -> h_h2x/1
  Qp2a,v5/1 -> Mux3/1, Mux4/1
  h_h2x/1 -> Mux4/2
  veh spd/1 -> Va/Vv/1, Mux5/2, Va/Vv1/1
  Va/Vv/1 -> Mux3/2
  Qi2c,c/1 -> Qfc_c/1, Qi/1
  fc_temp/1 -> Qx2p,c/1, Qh2x,r/1, Qp2a,v7/1, Qp2a,v6/1, Qh2a,r/1, Qh2x,r1/1, Qp2a,v5/1, Qx2i,c/1, Qi2c,c/1
  Qx2i,c/1 -> Qi/2, Qx/1
  Qi/1 -> Qfc_i/1
  Qx/1 -> Qfc_x/1
  Qh2x/1 -> Qx/2, Qh/1
  Qh/1 -> Qfc_h/1
  Mux6/1 -> Qh2a,v/1
  Mux5/1 -> h_h2a/1
  Qp2a,v6/1 -> Mux5/1, Mux6/1
  h_h2a/1 -> Mux6/2
  Qx1/1 -> Qx/3
  Qh2x,v/1 -> Qh2x/2
  Qx2p,c/1 -> Qh2x/1
  Qh2x,r1/1 -> Qx1/2
  Qh2x,v1/1 -> Qx1/1
  Qh2a,r/1 -> Qh/3
  Qh2a,v/1 -> Qh/2
  Qh2x,r/1 -> Qh2x/3

== system lib_fuel_converter3/configurable subsystems/fuel use and EO emis/fc temp/old fc coolant  temp. (C) ==
  fc on? : Inport
  veh spd : Inport  Port=2
  Block NOTES : Subsystem
      mask Display: disp('Block\nNOTES')
  Mux : Mux
  TEC : Integrator  InitialCondition=fc_i_init_tmp
  compute engine dT/dt : Fcn  Expr=1.1*u[1]*(-u[2]/218)*(95-u[4])+(1-u[1])*u[3]*(u[4]-amb_tmp)
  gamma (takes v as input) : Fcn  Expr=(-8.22e-5*u+8.09e-6*4-1.45e-4)*.45
  log(1-40/75) : Constant  Value=-0.7621
  fc coolant  temp (C) : Outport  InitialOutput=0
  wires:
  compute engine dT/dt/1 -> TEC/1
  gamma (takes v as input)/1 -> Mux/3
  log(1-40/75)/1 -> Mux/2
  Mux/1 -> compute engine dT/dt/1
  fc on?/1 -> Mux/1
  veh spd/1 -> gamma (takes v as input)/1
  TEC/1 -> fc coolant  temp (C)/1, Mux/4

== system lib_fuel_converter3/configurable subsystems/fuel use and EO emis/fc temp correct/fc temp correct Constant Correction Factors (Equation Based) ==
  Coolant T (C) : Inport
  HOT fuel use (g/s) : Inport  Port=2
  HOT emis (g/s) : Inport  Port=3
  Enable : EnablePort  StatesWhenEnabling=reset
  Block NOTES : Subsystem
      mask Display: disp('Block\nNOTES')
  CO cold/hot : Fcn  Expr=2.13*pow(u,4.26)+1
  HC cold/hot : Fcn  Expr=8.05*pow(u,9.46)+1
  Mux : Mux
  NOx cold/hot : Fcn  Expr=0.51*pow(u,1.37)+1
  PM cold/hot : Fcn  Expr=5.14*pow(u,17.04)+1
  Product : Product  SaturateOnIntegerOverflow=on
  Product1 : Product  SaturateOnIntegerOverflow=on
  Saturation : Saturate  UpperLimit=1  LowerLimit=0
  fuel cold/hot : Fcn  Expr=0.1*pow(u,0.65)+1
  lambda : Fcn  Expr=(fc_tstat-u)/(fc_tstat-20)
  fuel use (g/s) : Outport  OutputWhenDisabled=reset  InitialOutput=0
  EO emis (g/s) : Outport  Port=2  OutputWhenDisabled=reset  InitialOutput=0
  wires:
  PM cold/hot/1 -> Mux/4
  NOx cold/hot/1 -> Mux/3
  HC cold/hot/1 -> Mux/1
  Saturation/1 -> CO cold/hot/1, HC cold/hot/1, fuel cold/hot/1, NOx cold/hot/1, PM cold/hot/1
  lambda/1 -> Saturation/1
  Mux/1 -> Product/1
  fuel cold/hot/1 -> Product1/2
  Product/1 -> EO emis (g/s)/1
  CO cold/hot/1 -> Mux/2
  Product1/1 -> fuel use (g/s)/1
  HOT fuel use (g/s)/1 -> Product1/1
  Coolant T (C)/1 -> lambda/1
  HOT emis (g/s)/1 -> Product/2
